simulink model "linear_bicycle_model"  (R2023b)
settings: Solver=VariableStepAuto  StartTime=0.0  StopTime=10  RelTol=1e-3
libraries: autolibshared x1
settings Model: Creator=bglen  LastModifiedBy=bglen

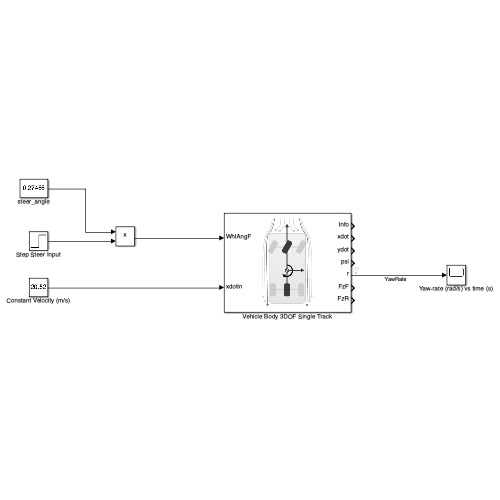
[thumbnail: Simulink's stored preview of the top-level diagram]
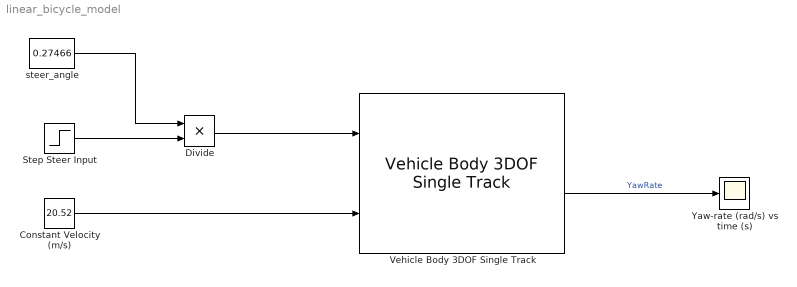
== system linear_bicycle_model ==
  Constant Velocity (m/s) : Constant  Value=20.52
  Divide : Product  Inputs=**
  Step Steer Input : Step  SampleTime=0
  Vehicle Body 3DOF Single Track : autolibshared/Vehicle Body 3DOF Single Track  trackMode=Single (bicycle)  inputMode=External longitudinal velocity  frontSteerMode=on  rearSteerMode=off  windMode=off  muMode=off  extFMode=off  extMMode=off  htchFMode=off  htchMMode=off  extXo=off  extpsio=off  extxdoto=off  extro=off  extYo=off  extTamb=off  extydoto=off  aMode=2  NF=2  NR=2  m=280  a=0.7956  b=0.7344  h=0.001  dh=1  hh=0.2  X_o=0  xdot_o=0  CalphaMode=off  sigmaMode=off  d=0  hl=0  w=[1.4,1.4]  Cy_f=28648  Cy_r=28648  sigma_f=.1  sigma_r=.1  alpha_f_brk=[-.1 .1]  Cy_f_data=[-9e3 9e3]  alpha_r_brk=[-.1 .1]  Cy_r_data=[-9e3 9e3]  Y_o=0  ydot_o=0  Izz=80  psi_o=0  r_o=0  Af=1.5  Cd=.3  Cl=.1  Cpm=.1  beta_w=[0 0.01:0.01:0.3]  Cs=[0 0.01:0.01:0.3]  Cym=[0 1e-6:0.01:0.3]  Pabs=101325  Tair=273  g=9.81  mu=1  xdot_tol=.01  Fznom=2746.8  Fxtire_sat=7e4  Fytire_sat=7e4  longOff=0  latOff=0  vertOff=0  wrapAng=off
  Yaw-rate (rad/s) vs time (s) : Scope
  steer_angle : Constant  Value=0.27466
  wires:
  Constant Velocity (m/s)/1 -> Vehicle Body 3DOF Single Track/2
  Divide/1 -> Vehicle Body 3DOF Single Track/1
  Step Steer Input/1 -> Divide/2
  steer_angle/1 -> Divide/1
  Vehicle Body 3DOF Single Track/5 -> Yaw-rate (rad/s) vs time (s)/1  "YawRate"
